simulink model "bot_sim_interface"  (R2018a)
settings: Solver=VariableStepAuto  StartTime=0.0  StopTime=inf  RelTol=1e-3
settings Model: Creator=Hussam  LastModifiedBy=hp 450

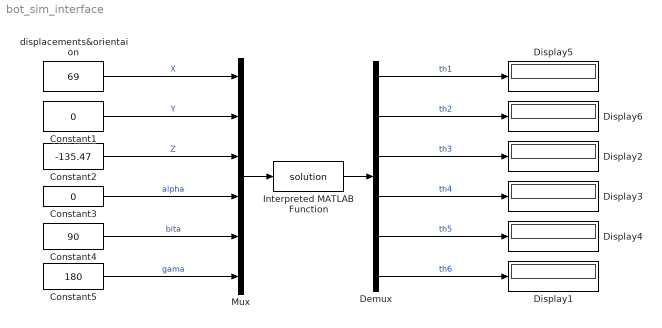
== system bot_sim_interface ==
  Constant1 : Constant  Value=0
  Constant2 : Constant  Value=-135.47
  Constant3 : Constant  Value=0
  Constant4 : Constant  Value=90
  Constant5 : Constant  Value=180
  Demux : Demux  Outputs=6
  Display{1..6} (6 alike) : Display
  Interpreted MATLAB Function : MATLABFcn  MATLABFcn=solution  OutputDimensions=6  OutputSignalType=complex
  Mux : Mux  Inputs=6
  displacements&orientaion : Constant  Value=69
  wires:
  Constant5/1 -> Mux/6  "gama"
  Constant4/1 -> Mux/5  "bita"
  Constant3/1 -> Mux/4  "alpha"
  Constant2/1 -> Mux/3  "Z"
  Constant1/1 -> Mux/2  "Y"
  displacements&orientaion/1 -> Mux/1  "X"
  Demux/6 -> Display1/1  "th6"
  Demux/5 -> Display4/1  "th5"
  Demux/4 -> Display3/1  "th4"
  Demux/1 -> Display5/1  "th1"
  Demux/2 -> Display6/1  "th2"
  Demux/3 -> Display2/1  "th3"
  Interpreted MATLAB Function/1 -> Demux/1
  Mux/1 -> Interpreted MATLAB Function/1
